simulink model "Simulink_Funktionsblock"  (R2019b)
settings: Solver=VariableStepAuto  StartTime=0.0  StopTime=3000  RelTol=1e-3
values from neighbouring files (symbols this model uses):
  A = double(subs(subs(subs( jacobian(dx_dt,vec_x), vec_x, x_AP), vec_e, e_AP), vec_u, u_AP))    [Modellbildung_Startbrenner.m]
  B = double(subs(subs(subs( jacobian(dx_dt,vec_u), vec_x, x_AP), vec_e, e_AP), vec_u, u_AP))    [Modellbildung_Startbrenner.m]
  B_e = [B,E]    [Modellbildung_Startbrenner.m]
  C = [1,0,0;0,1,0;0,0,1]    [Modellbildung_Startbrenner.m]
  C_lin = [1,0,0;0,1,0]    [Modellbildung_Startbrenner.m]
  D_e = zeros(3,5)    [Modellbildung_Startbrenner.m]
  D_lin = zeros(2,2)    [Modellbildung_Startbrenner.m]
  e_AP = [T_bg_in ; T_wt_in ; T_u]    [Modellbildung_Startbrenner.m]
  K = place(A,B,p_w)    [Modellbildung_Startbrenner.m]
  K_e = place(A,B_e,p_w)    [Modellbildung_Startbrenner.m]
  Par_Ini = [ 293.15  ; 293.15 ; 293.15  ]    [Modellbildung_Startbrenner.m]
  Par_Ini_lin = Par_Ini - x_AP    [Modellbildung_Startbrenner.m]
  S = (C_lin*((B*K-A)^(-1))*B)^(-1)    [Modellbildung_Startbrenner.m]
  u_AP = [ ms_bg ; ms_wt_air ]    [Modellbildung_Startbrenner.m]
  vec_par = zeros(19,1)    [Modellbildung_Startbrenner.m]
  x_AP = [double(x_AP_berechnet.x1) ; double(x_AP_berechnet.x2) ; double(x_AP_berechnet.x3)]    [Modellbildung_Startbrenner.m]
  x_AP_lin = [double(x_AP_berechnet.x1) ; double(x_AP_berechnet.x2) ]    [Modellbildung_Startbrenner.m]
  x_soll = [ 2400 ; 2000]    [Modellbildung_Startbrenner.m]
settings Model: Creator=mh981  LastModifiedBy=michael
settings DataIOCC: ReturnWorkspaceOutputs=off
settings DebuggingCC: ArithmeticOperatorsInVariantConditions=warning
settings SFSimCC: CustomCodeUndefinedFunction=UseInterfaceOnly

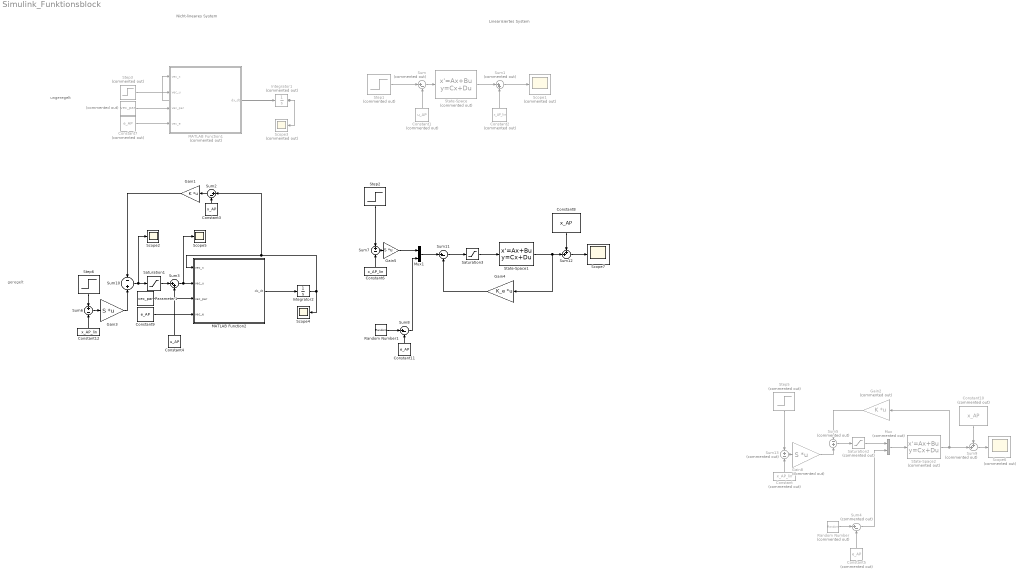
== system Simulink_Funktionsblock ==
  note: ungeregelt
  note: Linearisiertes System
  note: Nicht-lineares System
  note: geregelt
  " " : Constant  Commented=on  Value=vec_par
  Constant : Constant  Commented=on  Value=x_AP_lin
  Constant1 : Constant  Commented=on  Value=u_AP
  Constant10 : Constant  Commented=on  Value=x_AP
  Constant11 : Constant  Value=e_AP
  Constant12 : Constant  Value=x_AP_lin
  Constant2 : Constant  Commented=on  Value=x_AP_lin
  Constant3 : Constant  Value=x_AP
  Constant4 : Constant  Value=u_AP
  Constant5 : Constant  Commented=on  Value=e_AP
  Constant6 : Constant  Value=x_AP_lin
  Constant7 : Constant  Commented=on  Value=e_AP
  Constant8 : Constant  Value=x_AP
  Constant9 : Constant  Value=e_AP
  Gain1 : Gain  Gain=K  Multiplication=Matrix(K*u) (u vector)
  Gain2 : Gain  Commented=on  Gain=K  Multiplication=Matrix(K*u) (u vector)
  Gain3 : Gain  Gain=S  Multiplication=Matrix(K*u) (u vector)
  Gain4 : Gain  Gain=K_e  Multiplication=Matrix(K*u) (u vector)
  Gain5 : Gain  Gain=S  Multiplication=Matrix(K*u)
  Gain8 : Gain  Commented=on  Gain=S  Multiplication=Matrix(K*u) (u vector)
  Integrator1 : Integrator  Commented=on  InitialCondition=Par_Ini
  Integrator2 : Integrator  InitialCondition=Par_Ini
  MATLAB Function1 : MATLAB Function  Commented=on  TreatAsAtomicUnit=on
  MATLAB Function2 : MATLAB Function  TreatAsAtomicUnit=on
  Mux : Mux  Commented=on  Inputs=2
  Mux1 : Mux  Inputs=2
  Parameter1 : Constant  Value=vec_par
  Random Number : RandomNumber  Commented=on  Mean=e_AP  Variance=25  SampleTime=0.1
  Random Number1 : RandomNumber  Mean=e_AP  Variance=25  SampleTime=0.1
  Saturation1 : Saturate  UpperLimit=Inf  LowerLimit=0
  Saturation2 : Saturate  Commented=on  UpperLimit=Inf  LowerLimit=0
  Saturation3 : Saturate  UpperLimit=Inf  LowerLimit=0
  Scope1 : Scope  Commented=on
  Scope{2,4..5,7} (4 alike) : Scope
  Scope3 : Scope  Commented=on
  Scope6 : Scope  Commented=on
  State-Space : StateSpace  Commented=on  A=A  B=B  C=C_lin  D=D_lin  InitialCondition=Par_Ini_lin
  State-Space1 : StateSpace  A=A  B=B_e  C=C  D=D_e  InitialCondition=Par_Ini_lin
  State-Space2 : StateSpace  Commented=on  A=A  B=B_e  C=C  D=D_e  InitialCondition=Par_Ini_lin
  Step1 : Step  Commented=on  Time=0  Before=u_AP  After=u_AP  SampleTime=0
  Step2 : Step  Time=0  Before=x_soll  After=x_soll  SampleTime=0
  Step3 : Step  Commented=on  Time=0  Before=u_AP  After=u_AP  SampleTime=0
  Step5 : Step  Commented=on  Time=0  Before=x_soll  After=x_soll  SampleTime=0
  Step6 : Step  Time=0  Before=x_soll  After=x_soll  SampleTime=0
  Sum : Sum  Commented=on  Inputs=|+-
  Sum1 : Sum  Commented=on  Inputs=|++
  Sum10 : Sum  Inputs=-|+
  Sum11 : Sum  Inputs=|+-
  Sum12 : Sum  Inputs=++|
  Sum13 : Sum  Commented=on  Inputs=+|-
  Sum2 : Sum  Inputs=|+-
  Sum3 : Sum  Inputs=|++
  Sum4 : Sum  Commented=on  Inputs=|+-
  Sum5 : Sum  Commented=on  Inputs=-|+
  Sum6 : Sum  Inputs=+|-
  Sum7 : Sum  Inputs=+|-
  Sum8 : Sum  Inputs=|+-
  Sum9 : Sum  Commented=on  Inputs=++|
  wires:
  Sum1/1 -> Scope1/1
  State-Space/1 -> Sum1/1
  Constant1/1 -> Sum/2
  Constant2/1 -> Sum1/2
  Step1/1 -> Sum/1
  Sum/1 -> State-Space/1
  MATLAB Function1/1(dx_dt) -> Integrator1/1
  " "/1 -> MATLAB Function1/3(vec_par)
  Integrator1/1 -> Scope3/1, MATLAB Function1/1(vec_x)
  Constant7/1 -> MATLAB Function1/4(vec_e)
  Step3/1 -> MATLAB Function1/2(vec_u)
  Constant9/1 -> MATLAB Function2/4(vec_e)
  MATLAB Function2/1(dx_dt) -> Integrator2/1
  Parameter1/1 -> MATLAB Function2/3(vec_par)
  Sum10/1 -> Scope2/1, Saturation1/1
  Gain1/1 -> Sum10/1
  Constant10/1 -> Sum9/1
  Step5/1 -> Sum13/1
  Gain8/1 -> Sum5/2
  Sum13/1 -> Gain8/1
  Constant/1 -> Sum13/2
  Gain2/1 -> Sum5/1
  Sum6/1 -> Gain3/1
  Constant12/1 -> Sum6/2
  Step6/1 -> Sum6/1
  Gain3/1 -> Sum10/2
  Constant3/1 -> Sum2/2
  Integrator2/1 -> Scope4/1, Sum2/1, MATLAB Function2/1(vec_x)
  Sum2/1 -> Gain1/1
  Sum9/1 -> Scope6/1
  Constant4/1 -> Sum3/2
  Saturation1/1 -> Sum3/1
  Sum3/1 -> Scope5/1, MATLAB Function2/2(vec_u)
  State-Space2/1 -> Sum9/2, Gain2/1
  Random Number/1 -> Sum4/1
  Constant5/1 -> Sum4/2
  Sum4/1 -> Mux/2
  Sum5/1 -> Saturation2/1
  Saturation2/1 -> Mux/1
  Mux/1 -> State-Space2/1
  Gain4/1 -> Sum11/2
  Step2/1 -> Sum7/1
  Constant11/1 -> Sum8/2
  State-Space1/1 -> Sum12/2, Gain4/1
  Random Number1/1 -> Sum8/1
  Gain5/1 -> Mux1/1
  Saturation3/1 -> State-Space1/1
  Sum8/1 -> Mux1/2
  Constant8/1 -> Sum12/1
  Sum12/1 -> Scope7/1
  Constant6/1 -> Sum7/2
  Sum7/1 -> Gain5/1
  Sum11/1 -> Saturation3/1
  Mux1/1 -> Sum11/1

== matlab function Simulink_Funktionsblock/MATLAB Function1 ==
  data: vec_x input; vec_u input; dx_dt output; vec_par input; vec_e input
%#eml
function dx_dt = Modell_simulink(vec_x ,vec_u , vec_par , vec_e)

dx_dt = Modellgleichung_Startbrenner (vec_x ,vec_u , vec_par , vec_e);

== matlab function Simulink_Funktionsblock/MATLAB Function2 ==
  data: vec_x input; vec_u input; dx_dt output; vec_par input; vec_e input
%#eml
function dx_dt = Modell_simulink(vec_x ,vec_u , vec_par , vec_e)

dx_dt = Modellgleichung_Startbrenner (vec_x ,vec_u , vec_par , vec_e);
